simulink model "DOG_X_integer_true_two_paths_5b"  (R2024a)
settings: Solver=ode45  StartTime=0.0  StopTime=1.5*lsim*Ts  MaxStep=1/f0/2  RelTol=1e-6
values from neighbouring files (symbols this model uses):
  ft = (bint-1)*fbin    [exe_DOG_X_bit_true_2023a.m]    (also in exe_DOG_X_integer_true_two_paths_5b.m)
  g1 = g1_ideal*1    (= 4)    [exe_DOG_X_bit_true_2023a.m]    (also in exe_DOG_X_integer_true_two_paths_5b.m)
  Kvco = f0    (= 99840000)    [exe_DOG_X_bit_true_2023a.m]    (also in exe_DOG_X_integer_true_two_paths_5b.m)
  lvl = Vfs*10^(Input_signal_dB/20)    (= 0.125892541179)    [exe_DOG_X_bit_true_2023a.m]    (also in exe_DOG_X_integer_true_two_paths_5b.m)
  Nbsv1 = Nbvco+4    (= 9)    [exe_DOG_X_bit_true_2023a.m]    (also in exe_DOG_X_integer_true_two_paths_5b.m)
  Nbsv2 = Nbsv1+Nbext    [exe_DOG_X_bit_true_2023a.m]    (also in exe_DOG_X_integer_true_two_paths_5b.m)
  pnoi = 10^(-(60)/10)*(Vfs^2/2)    (= 5e-07)    [exe_DOG_X_bit_true_2023a.m]    (also in exe_DOG_X_integer_true_two_paths_5b.m)
  T2 = 1/f2    (= 4.06901041667e-08)    [exe_DOG_X_bit_true_2023a.m]    (also in exe_DOG_X_integer_true_two_paths_5b.m)
  Ts = 1/fs    (= 3.25520833333e-07)    [exe_DOG_X_bit_true_2023a.m]    (also in exe_DOG_X_integer_true_two_paths_5b.m)
  Tslow = 1/fslow    (= 6.51041666667e-07)    [exe_DOG_X_bit_true_2023a.m]    (also in exe_DOG_X_integer_true_two_paths_5b.m)
  Vfs = 1    [exe_DOG_X_bit_true_2023a.m]    (also in exe_DOG_X_integer_true_two_paths_5b.m)
undefined symbols (not defined in the file or in its folder): fa, fb, fti
libraries: simulink_extras x99, simulink x8
(part 1 of 4)
settings Model: SimulationMode=accelerator  Creator=lhernandez  LastModifiedBy=tremo
settings DataIOCC: SaveOutput=off  SignalLogging=off  DSMLogging=off  SaveTime=off  ReturnWorkspaceOutputs=off
settings RTWCC: GPUComputeCapability=3.5

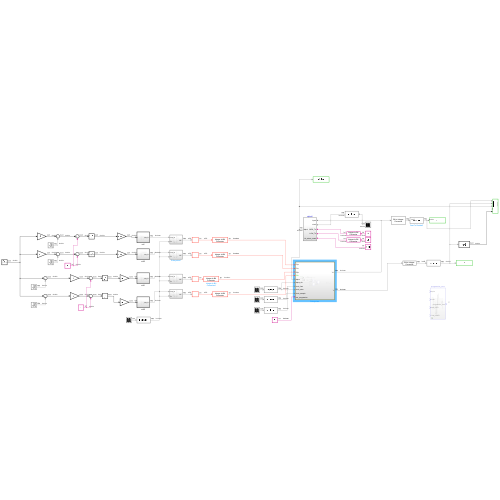
[thumbnail: Simulink's stored preview of the top-level diagram]
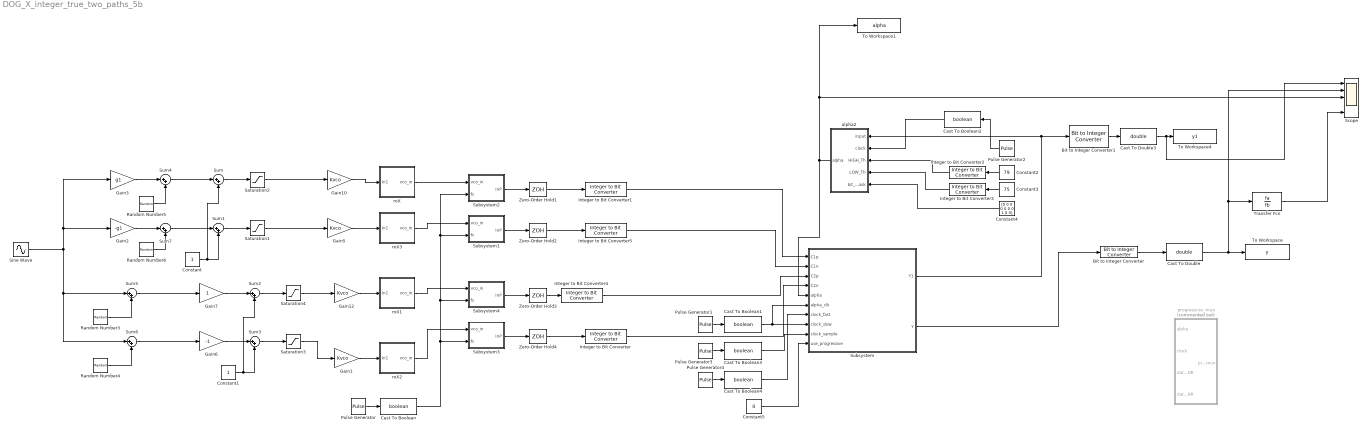
== system DOG_X_integer_true_two_paths_5b ==
  Bit to Integer Converter : simulink/Logic and Bit Operations/Bit to Integer Converter  nbits=11  bitOrder=MSB first  signedOutputValues=Signed  outDtype=Inherit via internal rule  outDtypeSigned=Inherit via internal rule
  Bit to Integer Converter1 : simulink/Logic and Bit Operations/Bit to Integer Converter  nbits=9  bitOrder=MSB first  signedOutputValues=Signed  outDtype=Inherit via internal rule  outDtypeSigned=Inherit via internal rule
  Cast To Boolean{,1..4} (5 alike) : DataTypeConversion  OutDataTypeStr=boolean  SaturateOnIntegerOverflow=off  RndMeth=Floor
  Cast To Double : DataTypeConversion  OutDataTypeStr=double  SaturateOnIntegerOverflow=off  RndMeth=Floor
  Cast To Double3 : DataTypeConversion  OutDataTypeStr=double  SaturateOnIntegerOverflow=off  RndMeth=Floor
  Constant : Constant
  Constant1 : Constant
  Constant2 : Constant  Value=79  OutDataTypeStr=fixdt(0,9,0)
  Constant3 : Constant  Value=75  OutDataTypeStr=fixdt(0,9,0)
  Constant4 : Constant  Value=[0 0 0 0 0 0 0 1 0 0]  OutDataTypeStr=boolean
  Constant5 : Constant  Value=0  OutDataTypeStr=boolean
  Gain{1,5,10,12} (4 alike) : Gain  Gain=Kvco
  Gain2 : Gain  Gain=-g1
  Gain3 : Gain  Gain=g1
  Gain6 : Gain  Gain=-1
  Gain7 : Gain
  Integer to Bit Converter{,1,4..5} (4 alike) : simulink/Logic and Bit Operations/Integer to Bit Converter  nbits=9  signedInputValues=Signed  bitOrder=MSB first  outDtype=boolean
  Integer to Bit Converter2 : simulink/Logic and Bit Operations/Integer to Bit Converter  nbits=9  signedInputValues=Unsigned  bitOrder=MSB first  outDtype=boolean
  Integer to Bit Converter3 : simulink/Logic and Bit Operations/Integer to Bit Converter  nbits=9  signedInputValues=Unsigned  bitOrder=MSB first  outDtype=boolean
  Pulse Generator : DiscretePulseGenerator  PulseType=Time based  Period=T2  PulseWidth=50
  Pulse Generator1 : DiscretePulseGenerator  PulseType=Time based  Period=Tslow  PulseWidth=50
  Pulse Generator2 : DiscretePulseGenerator  PulseType=Time based  Period=Tslow  PulseWidth=50
  Pulse Generator3 : DiscretePulseGenerator  PulseType=Time based  Period=Ts  PulseWidth=50
  Pulse Generator4 : DiscretePulseGenerator  PulseType=Time based  Period=T2  PulseWidth=50
  Random Number3 : RandomNumber  Variance=pnoi  Seed=35645  SampleTime=0
  Random Number4 : RandomNumber  Variance=pnoi  Seed=6854  SampleTime=0
  Random Number5 : RandomNumber  Variance=pnoi  Seed=5747  SampleTime=0
  Random Number6 : RandomNumber  Variance=pnoi  Seed=254745  SampleTime=0
  Saturation{1..4} (4 alike) : Saturate  UpperLimit=2  LowerLimit=0
  Scope : Scope  NumInputPorts=5
  Sine Wave : Sin  Amplitude=lvl/Vfs  Frequency=2*pi*ft  SampleTime=0
  Subsystem : Subsystem
  Subsystem1 : Subsystem
  Subsystem2 : Subsystem
  Subsystem3 : Subsystem
  Subsystem4 : Subsystem
  Sum{,1..7} (8 alike) : Sum  Inputs=|++
  To Workspace : ToWorkspace  VariableName=y  SampleTime=Ts
  To Workspace1 : ToWorkspace  VariableName=alpha  SampleTime=Ts
  To Workspace4 : ToWorkspace  VariableName=y1  SampleTime=Ts
  Transfer Fcn : TransferFcn  Numerator=fa  Denominator=fb
  Zero-Order Hold{1..4} (4 alike) : ZeroOrderHold  SampleTime=T2
  alpha2 : Subsystem
  progressive_mux : Subsystem  Commented=on
  roX : Subsystem
  roX1 : Subsystem
  roX2 : Subsystem
  roX3 : Subsystem
  wires:
  roX/1(vco_in) -> Subsystem2/1(vco_in)
  roX3/1(vco_in) -> Subsystem1/1(vco_in)
  Subsystem4/1(InP) -> Zero-Order Hold3/1
  Subsystem3/1(InP) -> Zero-Order Hold4/1
  Subsystem1/1(InP) -> Zero-Order Hold2/1
  Cast To Double/1 -> Transfer Fcn/1, Scope/2, To Workspace/1
  Cast To Double3/1 -> Scope/1, To Workspace4/1
  alpha2/1(alpha) -> Subsystem/5(alpha), To Workspace1/1, Scope/3
  Transfer Fcn/1 -> Scope/5
  Gain7/1 -> Sum2/1
  Saturation4/1 -> Gain12/1
  Sum5/1 -> Gain7/1
  Sum7/1 -> Sum1/1
  Gain10/1 -> roX/1(In1)
  Sum4/1 -> Sum/1
  Random Number6/1 -> Sum7/2
  Random Number4/1 -> Sum6/2
  Random Number3/1 -> Sum5/2
  Sine Wave/1 -> Sum6/1, Sum5/1, Gain3/1, Gain2/1
  Constant1/1 -> Sum2/2, Sum3/2
  Sum6/1 -> Gain6/1
  Sum/1 -> Saturation2/1
  Sum3/1 -> Saturation3/1
  Constant/1 -> Sum/2, Sum1/2
  Gain5/1 -> roX3/1(In1)
  Random Number5/1 -> Sum4/2
  Gain3/1 -> Sum4/1
  Gain2/1 -> Sum7/1
  Saturation3/1 -> Gain1/1
  Saturation2/1 -> Gain10/1
  Sum1/1 -> Saturation1/1
  Gain12/1 -> roX1/1(In1)
  Gain6/1 -> Sum3/1
  Sum2/1 -> Saturation4/1
  Saturation1/1 -> Gain5/1
  Gain1/1 -> roX2/1(In1)
  Subsystem2/1(InP) -> Zero-Order Hold1/1
  roX1/1(vco_in) -> Subsystem4/1(vco_in)
  roX2/1(vco_in) -> Subsystem3/1(vco_in)
  Zero-Order Hold3/1 -> Integer to Bit Converter4/1
  Zero-Order Hold4/1 -> Integer to Bit Converter/1
  Pulse Generator/1 -> Cast To Boolean/1
  Cast To Boolean/1 -> Subsystem3/2(fs), Subsystem4/2(fs), Subsystem1/2(fs), Subsystem2/2(fs)
  Subsystem/1(Y1) -> Bit to Integer Converter1/1, alpha2/1(input)
  Pulse Generator2/1 -> Cast To Boolean2/1
  Cast To Boolean2/1 -> alpha2/2(clock)
  Constant2/1 -> Integer to Bit Converter2/1
  Integer to Bit Converter2/1 -> alpha2/3(HIGH_Th)
  Constant3/1 -> Integer to Bit Converter3/1
  Integer to Bit Converter3/1 -> alpha2/4(LOW_Th)
  Constant4/1 -> alpha2/5(bit_select_mask)
  Bit to Integer Converter/1 -> Cast To Double/1
  Pulse Generator1/1 -> Cast To Boolean1/1
  Cast To Boolean1/1 -> Subsystem/8(clock_slow), Subsystem/6(alpha_clk)
  Integer to Bit Converter/1 -> Subsystem/4(C2n)
  Integer to Bit Converter4/1 -> Subsystem/3(C2p)
  Zero-Order Hold2/1 -> Integer to Bit Converter5/1
  Zero-Order Hold1/1 -> Integer to Bit Converter1/1
  Pulse Generator3/1 -> Cast To Boolean3/1
  Cast To Boolean3/1 -> Subsystem/9(clock_sample)
  Pulse Generator4/1 -> Cast To Boolean4/1
  Cast To Boolean4/1 -> Subsystem/7(clock_fast)
  Bit to Integer Converter1/1 -> Cast To Double3/1
  Integer to Bit Converter1/1 -> Subsystem/1(C1p)
  Integer to Bit Converter5/1 -> Subsystem/2(C1n)
  Subsystem/2(Y) -> Bit to Integer Converter/1
  Constant5/1 -> Subsystem/10(use_progressive)

== system DOG_X_integer_true_two_paths_5b/Subsystem ==
  C1p : Inport
  C1n : Inport  Port=2
  C2p : Inport  Port=3
  C2n : Inport  Port=4
  alpha : Inport  Port=5
  alpha_clk : Inport  Port=6
  clock_fast : Inport  Port=7
  clock_slow : Inport  Port=8
  clock_sample : Inport  Port=9
  use_progressive : Inport  Port=10
  " 2 bit arithmetic left shift" : Subsystem
  " 2 bit extension" : Subsystem
  2ND_Noise_Shaper_pipelined3 : Subsystem
  Noise_shaper1 : Subsystem
  Noise_shaper2 : Subsystem
  Terminator : Terminator
  mux : Subsystem
  mux1 : Subsystem
  progressive_mux : Subsystem
  substractor2 : Subsystem
  Y1 : Outport
  Y : Outport  Port=2
  wires:
  Noise_shaper2/2(Y1) -> Y1/1
  substractor2/1(Cmux1) -> 2ND_Noise_Shaper_pipelined3/1(Cmux1)
  C2p/1 -> Noise_shaper2/1(InP)
  C2n/1 -> Noise_shaper2/2(InN)
  alpha_clk/1 -> progressive_mux/4(clock)
  alpha/1 -> mux/3(alpha), progressive_mux/3(alpha)
  progressive_mux/1(progressive_mux) -> mux1/1(progressive)
  clock_fast/1 -> Noise_shaper1/3(clock_fast), Noise_shaper2/3(clock_fast)
  clock_slow/1 -> Noise_shaper1/4(clock_slow), Noise_shaper2/4(clock_slow)
  Noise_shaper2/1(Y) -> " 2 bit arithmetic left shift"/1(in)
  " 2 bit arithmetic left shift"/1(x4) -> mux/1(data_HDR), progressive_mux/1(data_HDR)
  clock_sample/1 -> Noise_shaper1/5(clock_sample), Noise_shaper2/5(clock_sample)
  " 2 bit extension"/1(extended) -> mux/2(data_HSNR), progressive_mux/2(data_HSNR)
  C1n/1 -> Noise_shaper1/2(InN)
  C1p/1 -> Noise_shaper1/1(InP)
  Noise_shaper1/1(Y) -> " 2 bit extension"/1(in)
  Noise_shaper1/2(Y1) -> Terminator/1
  mux/1(out) -> mux1/2(non_progressive)
  mux1/1(out) -> Y/1
  use_progressive/1 -> mux1/3(select)

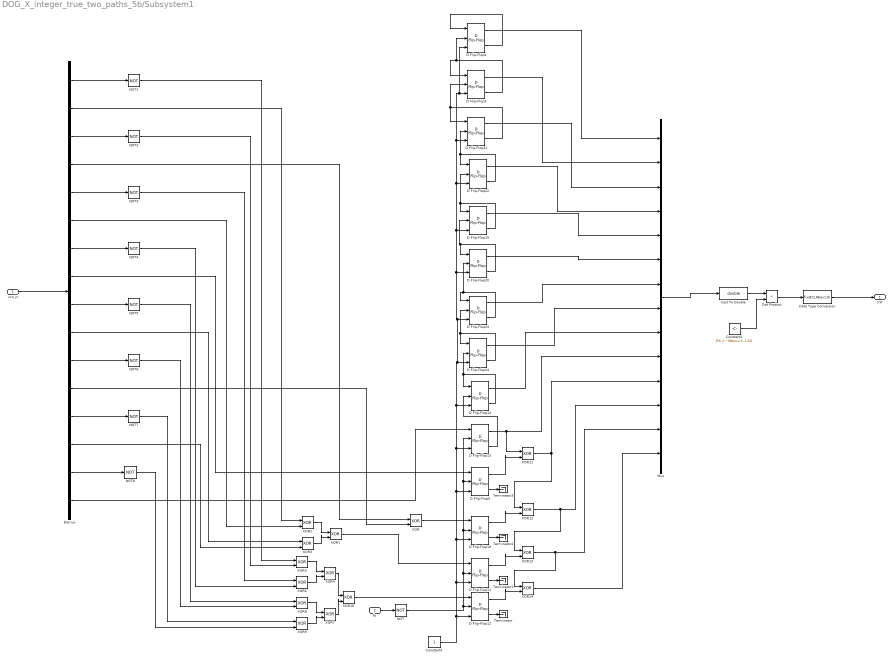
== system DOG_X_integer_true_two_paths_5b/Subsystem1 ==
  vco_in : Inport
  fs : Inport  Port=2
  Cast To Double : DataTypeConversion  OutDataTypeStr=double  SaturateOnIntegerOverflow=off  RndMeth=Floor
  Constant1 : Constant  Value=[fti 2.^(Nbsv1-1:-1:0)]
  Constant4 : Constant
  D Flip-Flop{3..4,9..15,20..24} (14 alike) : simulink_extras/Flip Flops/D Flip-Flop
  Data Type Conversion : DataTypeConversion  OutDataTypeStr=fixdt(1,Nbsv1,0)  SaturateOnIntegerOverflow=off  RndMeth=Floor
  Demux : Demux  Outputs=16
  Dot Product : DotProduct  OutDataTypeStr=Inherit: Inherit via internal rule
  Mux : Mux  Inputs=14
  NOT{,1..8} (9 alike) : Logic  Operator=NOT  IconShape=distinctive  AllPortsSameDT=off  OutDataTypeStr=boolean
  Terminator{,1..3} (4 alike) : Terminator
  XOR{,1..14} (15 alike) : Logic  Operator=XOR  IconShape=distinctive  AllPortsSameDT=off  OutDataTypeStr=boolean
  InP : Outport
  wires:
  D Flip-Flop12/2 -> Terminator/1
  D Flip-Flop10/2 -> Terminator2/1
  D Flip-Flop11/2 -> Terminator1/1
  D Flip-Flop22/2 -> D Flip-Flop21/2, D Flip-Flop22/1
  D Flip-Flop21/2 -> D Flip-Flop21/1, D Flip-Flop3/2
  D Flip-Flop23/2 -> D Flip-Flop20/2, D Flip-Flop23/1
  D Flip-Flop24/2 -> D Flip-Flop24/1, D Flip-Flop23/2
  D Flip-Flop20/2 -> D Flip-Flop15/2, D Flip-Flop20/1
  D Flip-Flop15/2 -> D Flip-Flop22/2, D Flip-Flop15/1
  Dot Product/1 -> Data Type Conversion/1
  Cast To Double/1 -> Dot Product/1
  Mux/1 -> Cast To Double/1
  fs/1 -> NOT/1
  D Flip-Flop14/2 -> D Flip-Flop14/1, D Flip-Flop24/2
  Constant1/1 -> Dot Product/2
  Data Type Conversion/1 -> InP/1
  Constant4/1 -> D Flip-Flop12/3, D Flip-Flop11/3, D Flip-Flop10/3, D Flip-Flop4/3, D Flip-Flop3/3, D Flip-Flop21/3, D Flip-Flop22/3, D Flip-Flop15/3, D Flip-Flop20/3, D Flip-Flop23/3, D Flip-Flop24/3, D Flip-Flop14/3, D Flip-Flop13/3, D Flip-Flop9/3
  D Flip-Flop13/2 -> D Flip-Flop14/2
  NOT/1 -> D Flip-Flop12/2, D Flip-Flop13/2, D Flip-Flop9/2, D Flip-Flop10/2, D Flip-Flop11/2
  D Flip-Flop3/2 -> D Flip-Flop4/2, D Flip-Flop3/1
  D Flip-Flop4/2 -> D Flip-Flop4/1
  D Flip-Flop4/1 -> Mux/1
  D Flip-Flop3/1 -> Mux/2
  D Flip-Flop21/1 -> Mux/3
  D Flip-Flop22/1 -> Mux/4
  D Flip-Flop15/1 -> Mux/5
  D Flip-Flop20/1 -> Mux/6
  D Flip-Flop23/1 -> Mux/7
  D Flip-Flop24/1 -> Mux/8
  D Flip-Flop14/1 -> Mux/9
  D Flip-Flop9/2 -> Terminator3/1
  vco_in/1 -> Demux/1
  Demux/1 -> NOT1/1
  Demux/5 -> NOT3/1
  Demux/7 -> NOT4/1
  Demux/9 -> NOT5/1
  Demux/13 -> NOT7/1
  Demux/15 -> NOT8/1
  Demux/11 -> NOT6/1
  Demux/4 -> XOR/1
  Demux/12 -> XOR/2
  XOR2/1 -> XOR1/1
  XOR3/1 -> XOR1/2
  Demux/2 -> XOR2/1
  Demux/6 -> XOR2/2
  Demux/10 -> XOR3/1
  Demux/14 -> XOR3/2
  XOR5/1 -> XOR4/1
  XOR6/1 -> XOR4/2
  XOR8/1 -> XOR7/1
  XOR9/1 -> XOR7/2
  XOR4/1 -> XOR10/1
  XOR7/1 -> XOR10/2
  Demux/3 -> NOT2/1
  D Flip-Flop13/1 -> XOR11/1, Mux/10
  D Flip-Flop9/1 -> XOR11/2
  XOR11/1 -> Mux/11, XOR12/1
  D Flip-Flop10/1 -> XOR12/2
  XOR12/1 -> XOR13/1, Mux/12
  D Flip-Flop11/1 -> XOR13/2
  XOR13/1 -> XOR14/1, Mux/13
  D Flip-Flop12/1 -> XOR14/2
  XOR14/1 -> Mux/14
  NOT1/1 -> XOR5/1
  NOT2/1 -> XOR5/2
  NOT3/1 -> XOR6/1
  NOT4/1 -> XOR6/2
  NOT5/1 -> XOR8/1
  NOT6/1 -> XOR8/2
  NOT7/1 -> XOR9/1
  NOT8/1 -> XOR9/2
  Demux/16 -> D Flip-Flop13/1
  Demux/8 -> D Flip-Flop9/1
  XOR/1 -> D Flip-Flop10/1
  XOR1/1 -> D Flip-Flop11/1
  XOR10/1 -> D Flip-Flop12/1

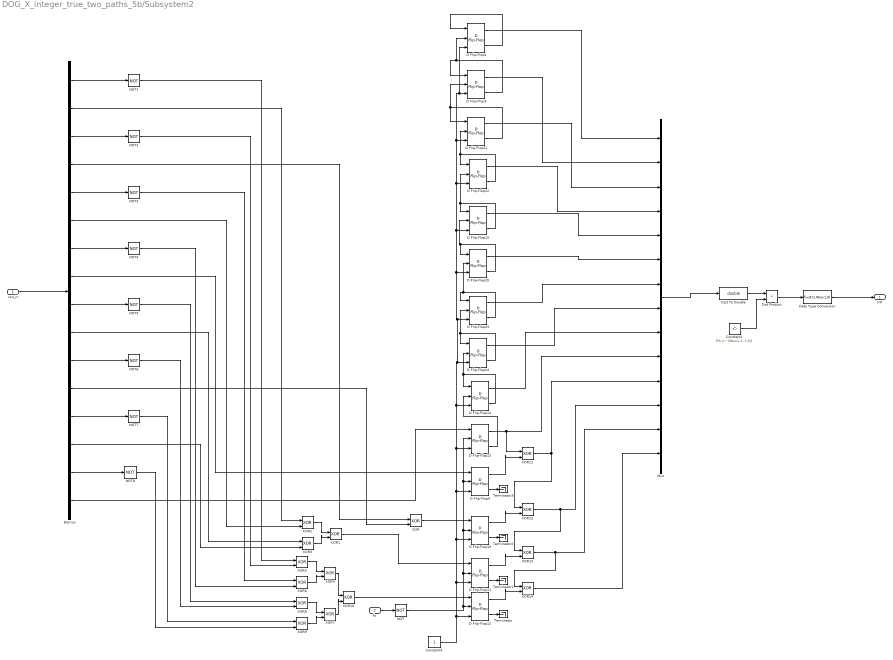
== system DOG_X_integer_true_two_paths_5b/Subsystem2 ==
  vco_in : Inport
  fs : Inport  Port=2
  Cast To Double : DataTypeConversion  OutDataTypeStr=double  SaturateOnIntegerOverflow=off  RndMeth=Floor
  Constant1 : Constant  Value=[fti 2.^(Nbsv1-1:-1:0)]
  Constant4 : Constant
  D Flip-Flop{3..4,9..15,20..24} (14 alike) : simulink_extras/Flip Flops/D Flip-Flop
  Data Type Conversion : DataTypeConversion  OutDataTypeStr=fixdt(1,Nbsv1,0)  SaturateOnIntegerOverflow=off  RndMeth=Floor
  Demux : Demux  Outputs=16
  Dot Product : DotProduct  OutDataTypeStr=Inherit: Inherit via internal rule
  Mux : Mux  Inputs=14
  NOT{,1..8} (9 alike) : Logic  Operator=NOT  IconShape=distinctive  AllPortsSameDT=off  OutDataTypeStr=boolean
  Terminator{,1..3} (4 alike) : Terminator
  XOR{,1..14} (15 alike) : Logic  Operator=XOR  IconShape=distinctive  AllPortsSameDT=off  OutDataTypeStr=boolean
  InP : Outport
  wires:
  D Flip-Flop12/2 -> Terminator/1
  D Flip-Flop10/2 -> Terminator2/1
  D Flip-Flop11/2 -> Terminator1/1
  D Flip-Flop22/2 -> D Flip-Flop21/2, D Flip-Flop22/1
  D Flip-Flop21/2 -> D Flip-Flop21/1, D Flip-Flop3/2
  D Flip-Flop23/2 -> D Flip-Flop20/2, D Flip-Flop23/1
  D Flip-Flop24/2 -> D Flip-Flop24/1, D Flip-Flop23/2
  D Flip-Flop20/2 -> D Flip-Flop15/2, D Flip-Flop20/1
  D Flip-Flop15/2 -> D Flip-Flop22/2, D Flip-Flop15/1
  Dot Product/1 -> Data Type Conversion/1
  Cast To Double/1 -> Dot Product/1
  Mux/1 -> Cast To Double/1
  fs/1 -> NOT/1
  D Flip-Flop14/2 -> D Flip-Flop14/1, D Flip-Flop24/2
  Constant1/1 -> Dot Product/2
  Data Type Conversion/1 -> InP/1
  Constant4/1 -> D Flip-Flop12/3, D Flip-Flop11/3, D Flip-Flop10/3, D Flip-Flop4/3, D Flip-Flop3/3, D Flip-Flop21/3, D Flip-Flop22/3, D Flip-Flop15/3, D Flip-Flop20/3, D Flip-Flop23/3, D Flip-Flop24/3, D Flip-Flop14/3, D Flip-Flop13/3, D Flip-Flop9/3
  D Flip-Flop13/2 -> D Flip-Flop14/2
  NOT/1 -> D Flip-Flop12/2, D Flip-Flop13/2, D Flip-Flop9/2, D Flip-Flop10/2, D Flip-Flop11/2
  D Flip-Flop3/2 -> D Flip-Flop4/2, D Flip-Flop3/1
  D Flip-Flop4/2 -> D Flip-Flop4/1
  D Flip-Flop4/1 -> Mux/1
  D Flip-Flop3/1 -> Mux/2
  D Flip-Flop21/1 -> Mux/3
  D Flip-Flop22/1 -> Mux/4
  D Flip-Flop15/1 -> Mux/5
  D Flip-Flop20/1 -> Mux/6
  D Flip-Flop23/1 -> Mux/7
  D Flip-Flop24/1 -> Mux/8
  D Flip-Flop14/1 -> Mux/9
  D Flip-Flop9/2 -> Terminator3/1
  vco_in/1 -> Demux/1
  Demux/1 -> NOT1/1
  Demux/5 -> NOT3/1
  Demux/7 -> NOT4/1
  Demux/9 -> NOT5/1
  Demux/13 -> NOT7/1
  Demux/15 -> NOT8/1
  Demux/11 -> NOT6/1
  Demux/4 -> XOR/1
  Demux/12 -> XOR/2
  XOR2/1 -> XOR1/1
  XOR3/1 -> XOR1/2
  Demux/2 -> XOR2/1
  Demux/6 -> XOR2/2
  Demux/10 -> XOR3/1
  Demux/14 -> XOR3/2
  XOR5/1 -> XOR4/1
  XOR6/1 -> XOR4/2
  XOR8/1 -> XOR7/1
  XOR9/1 -> XOR7/2
  XOR4/1 -> XOR10/1
  XOR7/1 -> XOR10/2
  Demux/3 -> NOT2/1
  D Flip-Flop13/1 -> XOR11/1, Mux/10
  D Flip-Flop9/1 -> XOR11/2
  XOR11/1 -> Mux/11, XOR12/1
  D Flip-Flop10/1 -> XOR12/2
  XOR12/1 -> XOR13/1, Mux/12
  D Flip-Flop11/1 -> XOR13/2
  XOR13/1 -> XOR14/1, Mux/13
  D Flip-Flop12/1 -> XOR14/2
  XOR14/1 -> Mux/14
  NOT1/1 -> XOR5/1
  NOT2/1 -> XOR5/2
  NOT3/1 -> XOR6/1
  NOT4/1 -> XOR6/2
  NOT5/1 -> XOR8/1
  NOT6/1 -> XOR8/2
  NOT7/1 -> XOR9/1
  NOT8/1 -> XOR9/2
  Demux/16 -> D Flip-Flop13/1
  Demux/8 -> D Flip-Flop9/1
  XOR/1 -> D Flip-Flop10/1
  XOR1/1 -> D Flip-Flop11/1
  XOR10/1 -> D Flip-Flop12/1

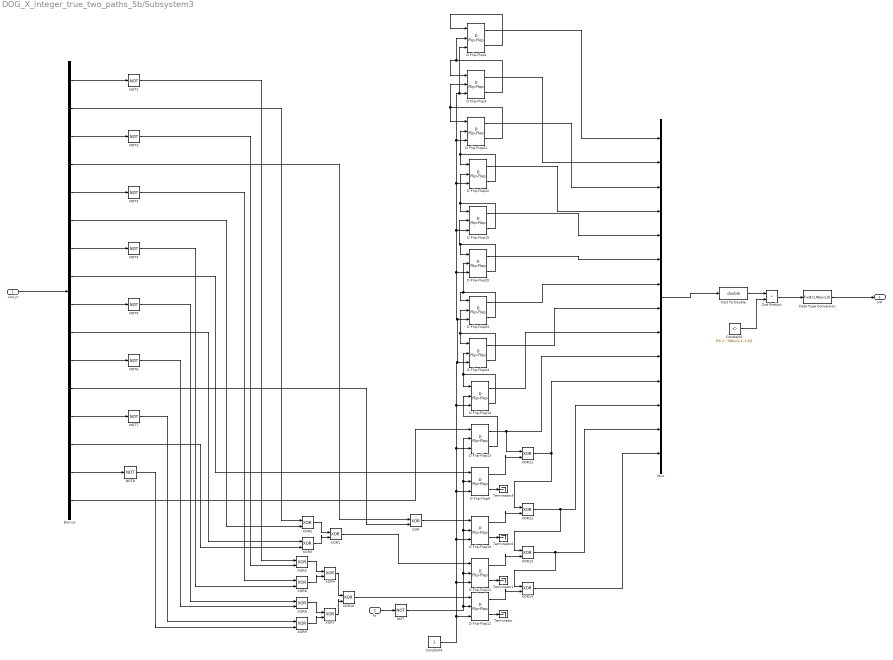
== system DOG_X_integer_true_two_paths_5b/Subsystem3 ==
  vco_in : Inport
  fs : Inport  Port=2
  Cast To Double : DataTypeConversion  OutDataTypeStr=double  SaturateOnIntegerOverflow=off  RndMeth=Floor
  Constant1 : Constant  Value=[fti 2.^(Nbsv1-1:-1:0)]
  Constant4 : Constant
  D Flip-Flop{3..4,9..15,20..24} (14 alike) : simulink_extras/Flip Flops/D Flip-Flop
  Data Type Conversion : DataTypeConversion  OutDataTypeStr=fixdt(1,Nbsv1,0)  SaturateOnIntegerOverflow=off  RndMeth=Floor
  Demux : Demux  Outputs=16
  Dot Product : DotProduct  OutDataTypeStr=Inherit: Inherit via internal rule
  Mux : Mux  Inputs=14
  NOT{,1..8} (9 alike) : Logic  Operator=NOT  IconShape=distinctive  AllPortsSameDT=off  OutDataTypeStr=boolean
  Terminator{,1..3} (4 alike) : Terminator
  XOR{,1..14} (15 alike) : Logic  Operator=XOR  IconShape=distinctive  AllPortsSameDT=off  OutDataTypeStr=boolean
  InP : Outport
  wires:
  D Flip-Flop12/2 -> Terminator/1
  D Flip-Flop10/2 -> Terminator2/1
  D Flip-Flop11/2 -> Terminator1/1
  D Flip-Flop22/2 -> D Flip-Flop21/2, D Flip-Flop22/1
  D Flip-Flop21/2 -> D Flip-Flop21/1, D Flip-Flop3/2
  D Flip-Flop23/2 -> D Flip-Flop20/2, D Flip-Flop23/1
  D Flip-Flop24/2 -> D Flip-Flop24/1, D Flip-Flop23/2
  D Flip-Flop20/2 -> D Flip-Flop15/2, D Flip-Flop20/1
  D Flip-Flop15/2 -> D Flip-Flop22/2, D Flip-Flop15/1
  Dot Product/1 -> Data Type Conversion/1
  Cast To Double/1 -> Dot Product/1
  Mux/1 -> Cast To Double/1
  fs/1 -> NOT/1
  D Flip-Flop14/2 -> D Flip-Flop14/1, D Flip-Flop24/2
  Constant1/1 -> Dot Product/2
  Data Type Conversion/1 -> InP/1
  Constant4/1 -> D Flip-Flop12/3, D Flip-Flop11/3, D Flip-Flop10/3, D Flip-Flop4/3, D Flip-Flop3/3, D Flip-Flop21/3, D Flip-Flop22/3, D Flip-Flop15/3, D Flip-Flop20/3, D Flip-Flop23/3, D Flip-Flop24/3, D Flip-Flop14/3, D Flip-Flop13/3, D Flip-Flop9/3
  D Flip-Flop13/2 -> D Flip-Flop14/2
  NOT/1 -> D Flip-Flop12/2, D Flip-Flop13/2, D Flip-Flop9/2, D Flip-Flop10/2, D Flip-Flop11/2
  D Flip-Flop3/2 -> D Flip-Flop4/2, D Flip-Flop3/1
  D Flip-Flop4/2 -> D Flip-Flop4/1
  D Flip-Flop4/1 -> Mux/1
  D Flip-Flop3/1 -> Mux/2
  D Flip-Flop21/1 -> Mux/3
  D Flip-Flop22/1 -> Mux/4
  D Flip-Flop15/1 -> Mux/5
  D Flip-Flop20/1 -> Mux/6
  D Flip-Flop23/1 -> Mux/7
  D Flip-Flop24/1 -> Mux/8
  D Flip-Flop14/1 -> Mux/9
  D Flip-Flop9/2 -> Terminator3/1
  vco_in/1 -> Demux/1
  Demux/1 -> NOT1/1
  Demux/5 -> NOT3/1
  Demux/7 -> NOT4/1
  Demux/9 -> NOT5/1
  Demux/13 -> NOT7/1
  Demux/15 -> NOT8/1
  Demux/11 -> NOT6/1
  Demux/4 -> XOR/1
  Demux/12 -> XOR/2
  XOR2/1 -> XOR1/1
  XOR3/1 -> XOR1/2
  Demux/2 -> XOR2/1
  Demux/6 -> XOR2/2
  Demux/10 -> XOR3/1
  Demux/14 -> XOR3/2
  XOR5/1 -> XOR4/1
  XOR6/1 -> XOR4/2
  XOR8/1 -> XOR7/1
  XOR9/1 -> XOR7/2
  XOR4/1 -> XOR10/1
  XOR7/1 -> XOR10/2
  Demux/3 -> NOT2/1
  D Flip-Flop13/1 -> XOR11/1, Mux/10
  D Flip-Flop9/1 -> XOR11/2
  XOR11/1 -> Mux/11, XOR12/1
  D Flip-Flop10/1 -> XOR12/2
  XOR12/1 -> XOR13/1, Mux/12
  D Flip-Flop11/1 -> XOR13/2
  XOR13/1 -> XOR14/1, Mux/13
  D Flip-Flop12/1 -> XOR14/2
  XOR14/1 -> Mux/14
  NOT1/1 -> XOR5/1
  NOT2/1 -> XOR5/2
  NOT3/1 -> XOR6/1
  NOT4/1 -> XOR6/2
  NOT5/1 -> XOR8/1
  NOT6/1 -> XOR8/2
  NOT7/1 -> XOR9/1
  NOT8/1 -> XOR9/2
  Demux/16 -> D Flip-Flop13/1
  Demux/8 -> D Flip-Flop9/1
  XOR/1 -> D Flip-Flop10/1
  XOR1/1 -> D Flip-Flop11/1
  XOR10/1 -> D Flip-Flop12/1

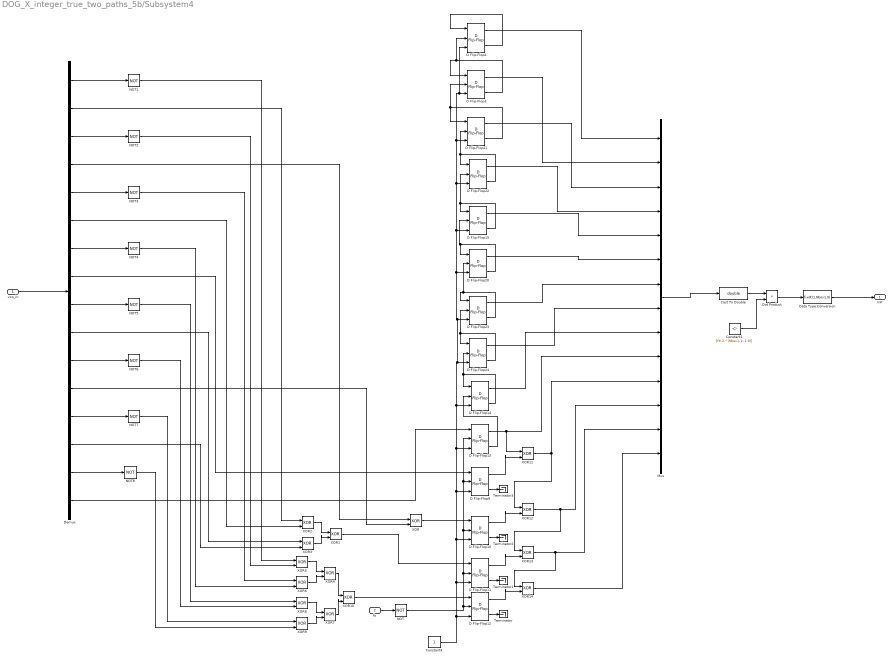
== system DOG_X_integer_true_two_paths_5b/Subsystem4 ==
  vco_in : Inport
  fs : Inport  Port=2
  Cast To Double : DataTypeConversion  OutDataTypeStr=double  SaturateOnIntegerOverflow=off  RndMeth=Floor
  Constant1 : Constant  Value=[fti 2.^(Nbsv1-1:-1:0)]
  Constant4 : Constant
  D Flip-Flop{3..4,9..15,20..24} (14 alike) : simulink_extras/Flip Flops/D Flip-Flop
  Data Type Conversion : DataTypeConversion  OutDataTypeStr=fixdt(1,Nbsv1,0)  SaturateOnIntegerOverflow=off  RndMeth=Floor
  Demux : Demux  Outputs=16
  Dot Product : DotProduct  OutDataTypeStr=Inherit: Inherit via internal rule
  Mux : Mux  Inputs=14
  NOT{,1..8} (9 alike) : Logic  Operator=NOT  IconShape=distinctive  AllPortsSameDT=off  OutDataTypeStr=boolean
  Terminator{,1..3} (4 alike) : Terminator
  XOR{,1..14} (15 alike) : Logic  Operator=XOR  IconShape=distinctive  AllPortsSameDT=off  OutDataTypeStr=boolean
  InP : Outport
  wires:
  D Flip-Flop12/2 -> Terminator/1
  D Flip-Flop10/2 -> Terminator2/1
  D Flip-Flop11/2 -> Terminator1/1
  D Flip-Flop22/2 -> D Flip-Flop21/2, D Flip-Flop22/1
  D Flip-Flop21/2 -> D Flip-Flop21/1, D Flip-Flop3/2
  D Flip-Flop23/2 -> D Flip-Flop20/2, D Flip-Flop23/1
  D Flip-Flop24/2 -> D Flip-Flop24/1, D Flip-Flop23/2
  D Flip-Flop20/2 -> D Flip-Flop15/2, D Flip-Flop20/1
  D Flip-Flop15/2 -> D Flip-Flop22/2, D Flip-Flop15/1
  Dot Product/1 -> Data Type Conversion/1
  Cast To Double/1 -> Dot Product/1
  Mux/1 -> Cast To Double/1
  fs/1 -> NOT/1
  D Flip-Flop14/2 -> D Flip-Flop14/1, D Flip-Flop24/2
  Constant1/1 -> Dot Product/2
  Data Type Conversion/1 -> InP/1
  Constant4/1 -> D Flip-Flop12/3, D Flip-Flop11/3, D Flip-Flop10/3, D Flip-Flop4/3, D Flip-Flop3/3, D Flip-Flop21/3, D Flip-Flop22/3, D Flip-Flop15/3, D Flip-Flop20/3, D Flip-Flop23/3, D Flip-Flop24/3, D Flip-Flop14/3, D Flip-Flop13/3, D Flip-Flop9/3
  D Flip-Flop13/2 -> D Flip-Flop14/2
  NOT/1 -> D Flip-Flop12/2, D Flip-Flop13/2, D Flip-Flop9/2, D Flip-Flop10/2, D Flip-Flop11/2
  D Flip-Flop3/2 -> D Flip-Flop4/2, D Flip-Flop3/1
  D Flip-Flop4/2 -> D Flip-Flop4/1
  D Flip-Flop4/1 -> Mux/1
  D Flip-Flop3/1 -> Mux/2
  D Flip-Flop21/1 -> Mux/3
  D Flip-Flop22/1 -> Mux/4
  D Flip-Flop15/1 -> Mux/5
  D Flip-Flop20/1 -> Mux/6
  D Flip-Flop23/1 -> Mux/7
  D Flip-Flop24/1 -> Mux/8
  D Flip-Flop14/1 -> Mux/9
  D Flip-Flop9/2 -> Terminator3/1
  vco_in/1 -> Demux/1
  Demux/1 -> NOT1/1
  Demux/5 -> NOT3/1
  Demux/7 -> NOT4/1
  Demux/9 -> NOT5/1
  Demux/13 -> NOT7/1
  Demux/15 -> NOT8/1
  Demux/11 -> NOT6/1
  Demux/4 -> XOR/1
  Demux/12 -> XOR/2
  XOR2/1 -> XOR1/1
  XOR3/1 -> XOR1/2
  Demux/2 -> XOR2/1
  Demux/6 -> XOR2/2
  Demux/10 -> XOR3/1
  Demux/14 -> XOR3/2
  XOR5/1 -> XOR4/1
  XOR6/1 -> XOR4/2
  XOR8/1 -> XOR7/1
  XOR9/1 -> XOR7/2
  XOR4/1 -> XOR10/1
  XOR7/1 -> XOR10/2
  Demux/3 -> NOT2/1
  D Flip-Flop13/1 -> XOR11/1, Mux/10
  D Flip-Flop9/1 -> XOR11/2
  XOR11/1 -> Mux/11, XOR12/1
  D Flip-Flop10/1 -> XOR12/2
  XOR12/1 -> XOR13/1, Mux/12
  D Flip-Flop11/1 -> XOR13/2
  XOR13/1 -> XOR14/1, Mux/13
  D Flip-Flop12/1 -> XOR14/2
  XOR14/1 -> Mux/14
  NOT1/1 -> XOR5/1
  NOT2/1 -> XOR5/2
  NOT3/1 -> XOR6/1
  NOT4/1 -> XOR6/2
  NOT5/1 -> XOR8/1
  NOT6/1 -> XOR8/2
  NOT7/1 -> XOR9/1
  NOT8/1 -> XOR9/2
  Demux/16 -> D Flip-Flop13/1
  Demux/8 -> D Flip-Flop9/1
  XOR/1 -> D Flip-Flop10/1
  XOR1/1 -> D Flip-Flop11/1
  XOR10/1 -> D Flip-Flop12/1

== system DOG_X_integer_true_two_paths_5b/alpha2 ==
  note: si a > b, reset
  note: si a > b, HDR
  input : Inport
  clock : Inport  Port=2
  HIGH_Th : Inport  Port=3
  LOW_Th : Inport  Port=4
  bit_select_mask : Inport  Port=5
  10 bit  counter (pos) : Subsystem
  AND : Logic  IconShape=distinctive  AllPortsSameDT=off  OutDataTypeStr=boolean
  AND1 : Logic  IconShape=distinctive  AllPortsSameDT=off  OutDataTypeStr=boolean
  NOT : Logic  Operator=NOT  IconShape=distinctive  AllPortsSameDT=off  OutDataTypeStr=boolean
  NOT1 : Logic  Operator=NOT  IconShape=distinctive  AllPortsSameDT=off  OutDataTypeStr=boolean
  NOT2 : Logic  Operator=NOT  IconShape=distinctive  AllPortsSameDT=off  OutDataTypeStr=boolean
  S-R Flip-Flop : simulink_extras/Flip Flops/S-R Flip-Flop  initial_condition=0
  Terminator : Terminator
  abs : Subsystem
  comp_HI_Threshold : Subsystem
  comp_LOW_Threshold : Subsystem
  alpha : Outport
  wires:
  input/1 -> abs/1(input)
  S-R Flip-Flop/1 -> alpha/1
  clock/1 -> 10 bit  counter (pos)/2(clock)
  LOW_Th/1 -> comp_LOW_Threshold/2(b)
  NOT1/1 -> 10 bit  counter (pos)/3(!reset)
  abs/1(abs(input)) -> comp_HI_Threshold/1(a), comp_LOW_Threshold/1(a)
  HIGH_Th/1 -> comp_HI_Threshold/2(b)
  S-R Flip-Flop/2 -> Terminator/1
  comp_LOW_Threshold/1(a < b) -> AND/2
  AND1/1 -> S-R Flip-Flop/2
  comp_HI_Threshold/1(a > b) -> NOT1/1, NOT2/1, S-R Flip-Flop/1
  NOT/1 -> AND/1
  NOT2/1 -> AND1/1
  10 bit  counter (pos)/1(count_selected_bit) -> AND1/2, NOT/1
  AND/1 -> 10 bit  counter (pos)/1(count_enable)
  bit_select_mask/1 -> 10 bit  counter (pos)/4(bit_select_mask)

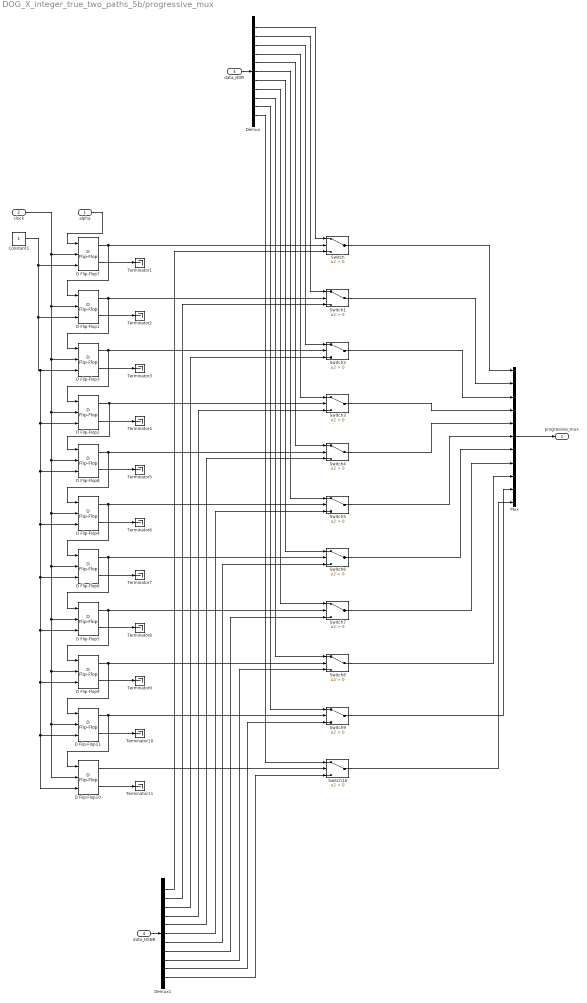
== system DOG_X_integer_true_two_paths_5b/progressive_mux ==
  alpha : Inport
  clock : Inport  Port=2
  data_HDR : Inport  Port=3
  data_HSNR : Inport  Port=4
  Constant1 : Constant  OutDataTypeStr=boolean
  D Flip-Flop{1..11} (11 alike) : simulink_extras/Flip Flops/D Flip-Flop
  Demux : Demux  Outputs=11
  Demux1 : Demux  Outputs=11
  Mux : Mux  Inputs=11
  Switch{,1..10} (11 alike) : Switch  Criteria=u2 > Threshold  SaturateOnIntegerOverflow=off  InputSameDT=off
  Terminator{1..11} (11 alike) : Terminator
  progressive_mux : Outport
  wires:
  D Flip-Flop7/1 -> Switch/2, D Flip-Flop1/1
  data_HDR/1 -> Demux/1
  data_HSNR/1 -> Demux1/1
  D Flip-Flop7/2 -> Terminator1/1
  D Flip-Flop1/2 -> Terminator2/1
  D Flip-Flop1/1 -> D Flip-Flop3/1, Switch1/2
  D Flip-Flop3/1 -> Switch2/2, D Flip-Flop2/1
  D Flip-Flop2/2 -> Terminator4/1
  D Flip-Flop3/2 -> Terminator3/1
  D Flip-Flop2/1 -> Switch3/2, D Flip-Flop8/1
  D Flip-Flop4/2 -> Terminator6/1
  D Flip-Flop8/1 -> Switch4/2, D Flip-Flop4/1
  D Flip-Flop6/2 -> Terminator7/1
  D Flip-Flop5/2 -> Terminator8/1
  D Flip-Flop6/1 -> Switch6/2, D Flip-Flop5/1
  D Flip-Flop8/2 -> Terminator5/1
  D Flip-Flop4/1 -> D Flip-Flop6/1, Switch5/2
  D Flip-Flop11/1 -> Switch9/2, D Flip-Flop10/1
  D Flip-Flop9/1 -> D Flip-Flop11/1, Switch8/2
  D Flip-Flop5/1 -> D Flip-Flop9/1, Switch7/2
  D Flip-Flop9/2 -> Terminator9/1
  D Flip-Flop11/2 -> Terminator10/1
  D Flip-Flop10/1 -> Switch10/2
  Constant1/1 -> D Flip-Flop8/3, D Flip-Flop10/3, D Flip-Flop11/3, D Flip-Flop9/3, D Flip-Flop5/3, D Flip-Flop6/3, D Flip-Flop4/3, D Flip-Flop2/3, D Flip-Flop3/3, D Flip-Flop1/3, D Flip-Flop7/3
  D Flip-Flop10/2 -> Terminator11/1
  clock/1 -> D Flip-Flop6/2, D Flip-Flop11/2, D Flip-Flop10/2, D Flip-Flop9/2, D Flip-Flop5/2, D Flip-Flop4/2, D Flip-Flop8/2, D Flip-Flop2/2, D Flip-Flop3/2, D Flip-Flop1/2, D Flip-Flop7/2
  alpha/1 -> D Flip-Flop7/1
  Demux/1 -> Switch/1
  Mux/1 -> progressive_mux/1
  Demux/2 -> Switch1/1
  Demux/3 -> Switch2/1
  Demux/4 -> Switch3/1
  Demux/5 -> Switch4/1
  Demux/6 -> Switch5/1
  Demux/7 -> Switch6/1
  Demux/8 -> Switch7/1
  Demux/9 -> Switch8/1
  Demux/10 -> Switch9/1
  Demux/11 -> Switch10/1
  Demux1/1 -> Switch/3
  Demux1/2 -> Switch1/3
  Demux1/3 -> Switch2/3
  Demux1/4 -> Switch3/3
  Demux1/5 -> Switch4/3
  Demux1/6 -> Switch5/3
  Demux1/7 -> Switch6/3
  Demux1/8 -> Switch7/3
  Demux1/9 -> Switch8/3
  Demux1/10 -> Switch9/3
  Demux1/11 -> Switch10/3
  Switch/1 -> Mux/1
  Switch1/1 -> Mux/2
  Switch2/1 -> Mux/3
  Switch3/1 -> Mux/4
  Switch4/1 -> Mux/5
  Switch5/1 -> Mux/6
  Switch6/1 -> Mux/7
  Switch7/1 -> Mux/8
  Switch8/1 -> Mux/9
  Switch9/1 -> Mux/10
  Switch10/1 -> Mux/11

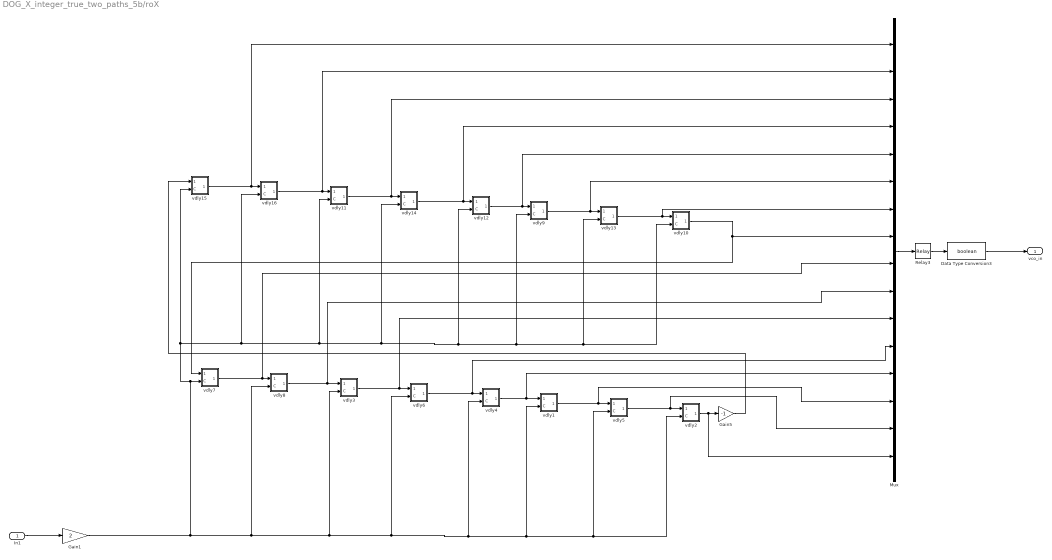
== system DOG_X_integer_true_two_paths_5b/roX ==
  In1 : Inport
  Data Type Conversion3 : DataTypeConversion  OutDataTypeStr=boolean  SaturateOnIntegerOverflow=off  RndMeth=Floor
  Gain1 : Gain  Gain=2
  Gain5 : Gain  Gain=-1
  Mux : Mux  Inputs=16
  Relay3 : Relay
  vdly1 : Subsystem
  vdly10 : Subsystem
  vdly11 : Subsystem
  vdly12 : Subsystem
  vdly13 : Subsystem
  vdly14 : Subsystem
  vdly15 : Subsystem
  vdly16 : Subsystem
  vdly2 : Subsystem
  vdly3 : Subsystem
  vdly4 : Subsystem
  vdly5 : Subsystem
  vdly6 : Subsystem
  vdly7 : Subsystem
  vdly8 : Subsystem
  vdly9 : Subsystem
  vco_in : Outport
  wires:
  vdly2/1(Out) -> Mux/16, Gain5/1
  In1/1 -> Gain1/1
  Gain1/1 -> vdly15/2(C), vdly16/2(C), vdly11/2(C), vdly14/2(C), vdly12/2(C), vdly9/2(C), vdly10/2(C), vdly13/2(C), vdly7/2(C), vdly8/2(C), vdly3/2(C), vdly6/2(C), vdly4/2(C), vdly1/2(C), vdly2/2(C), vdly5/2(C)
  Gain5/1 -> vdly15/1(In)
  Mux/1 -> Relay3/1
  Relay3/1 -> Data Type Conversion3/1
  Data Type Conversion3/1 -> vco_in/1
  vdly5/1(Out) -> Mux/15, vdly2/1(In)
  vdly1/1(Out) -> Mux/14, vdly5/1(In)
  vdly4/1(Out) -> Mux/13, vdly1/1(In)
  vdly6/1(Out) -> Mux/12, vdly4/1(In)
  vdly3/1(Out) -> Mux/11, vdly6/1(In)
  vdly8/1(Out) -> Mux/10, vdly3/1(In)
  vdly7/1(Out) -> vdly8/1(In), Mux/9
  vdly15/1(Out) -> Mux/1, vdly16/1(In)
  vdly16/1(Out) -> Mux/2, vdly11/1(In)
  vdly11/1(Out) -> Mux/3, vdly14/1(In)
  vdly14/1(Out) -> Mux/4, vdly12/1(In)
  vdly12/1(Out) -> Mux/5, vdly9/1(In)
  vdly9/1(Out) -> Mux/6, vdly13/1(In)
  vdly13/1(Out) -> Mux/7, vdly10/1(In)
  vdly10/1(Out) -> vdly7/1(In), Mux/8

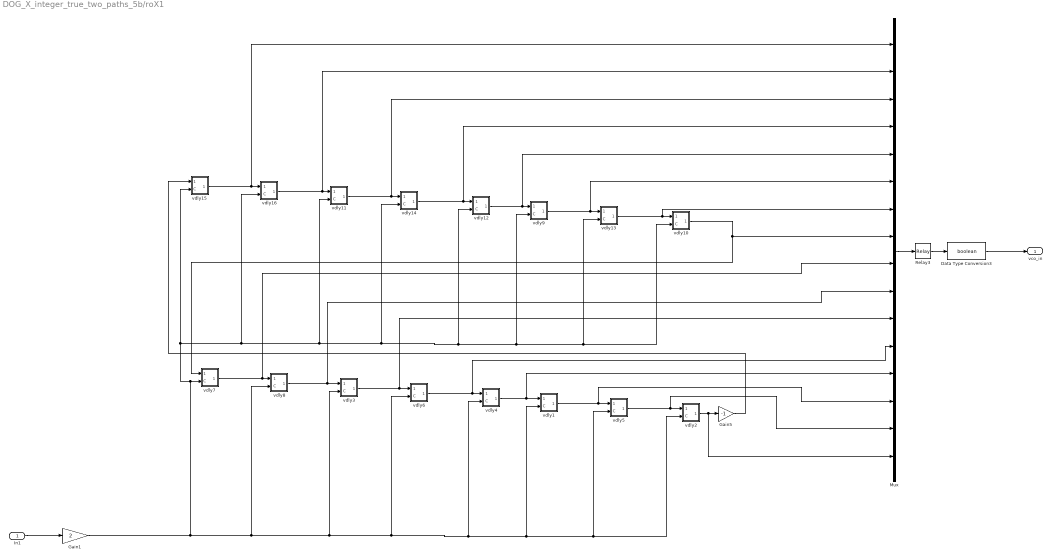
== system DOG_X_integer_true_two_paths_5b/roX1 ==
  In1 : Inport
  Data Type Conversion3 : DataTypeConversion  OutDataTypeStr=boolean  SaturateOnIntegerOverflow=off  RndMeth=Floor
  Gain1 : Gain  Gain=2
  Gain5 : Gain  Gain=-1
  Mux : Mux  Inputs=16
  Relay3 : Relay
  vdly1 : Subsystem
  vdly10 : Subsystem
  vdly11 : Subsystem
  vdly12 : Subsystem
  vdly13 : Subsystem
  vdly14 : Subsystem
  vdly15 : Subsystem
  vdly16 : Subsystem
  vdly2 : Subsystem
  vdly3 : Subsystem
  vdly4 : Subsystem
  vdly5 : Subsystem
  vdly6 : Subsystem
  vdly7 : Subsystem
  vdly8 : Subsystem
  vdly9 : Subsystem
  vco_in : Outport
  wires:
  vdly2/1(Out) -> Mux/16, Gain5/1
  In1/1 -> Gain1/1
  Gain1/1 -> vdly15/2(C), vdly16/2(C), vdly11/2(C), vdly14/2(C), vdly12/2(C), vdly9/2(C), vdly10/2(C), vdly13/2(C), vdly7/2(C), vdly8/2(C), vdly3/2(C), vdly6/2(C), vdly4/2(C), vdly1/2(C), vdly2/2(C), vdly5/2(C)
  Gain5/1 -> vdly15/1(In)
  Mux/1 -> Relay3/1
  Relay3/1 -> Data Type Conversion3/1
  Data Type Conversion3/1 -> vco_in/1
  vdly5/1(Out) -> Mux/15, vdly2/1(In)
  vdly1/1(Out) -> Mux/14, vdly5/1(In)
  vdly4/1(Out) -> Mux/13, vdly1/1(In)
  vdly6/1(Out) -> Mux/12, vdly4/1(In)
  vdly3/1(Out) -> Mux/11, vdly6/1(In)
  vdly8/1(Out) -> Mux/10, vdly3/1(In)
  vdly7/1(Out) -> vdly8/1(In), Mux/9
  vdly15/1(Out) -> Mux/1, vdly16/1(In)
  vdly16/1(Out) -> Mux/2, vdly11/1(In)
  vdly11/1(Out) -> Mux/3, vdly14/1(In)
  vdly14/1(Out) -> Mux/4, vdly12/1(In)
  vdly12/1(Out) -> Mux/5, vdly9/1(In)
  vdly9/1(Out) -> Mux/6, vdly13/1(In)
  vdly13/1(Out) -> Mux/7, vdly10/1(In)
  vdly10/1(Out) -> vdly7/1(In), Mux/8

== system DOG_X_integer_true_two_paths_5b/roX2 ==
  In1 : Inport
  Data Type Conversion3 : DataTypeConversion  OutDataTypeStr=boolean  SaturateOnIntegerOverflow=off  RndMeth=Floor
  Gain1 : Gain  Gain=2
  Gain5 : Gain  Gain=-1
  Mux : Mux  Inputs=16
  Relay3 : Relay
  vdly1 : Subsystem
  vdly10 : Subsystem
  vdly11 : Subsystem
  vdly12 : Subsystem
  vdly13 : Subsystem
  vdly14 : Subsystem
  vdly15 : Subsystem
  vdly16 : Subsystem
  vdly2 : Subsystem
  vdly3 : Subsystem
  vdly4 : Subsystem
  vdly5 : Subsystem
  vdly6 : Subsystem
  vdly7 : Subsystem
  vdly8 : Subsystem
  vdly9 : Subsystem
  vco_in : Outport
  wires:
  vdly2/1(Out) -> Mux/16, Gain5/1
  In1/1 -> Gain1/1
  Gain1/1 -> vdly15/2(C), vdly16/2(C), vdly11/2(C), vdly14/2(C), vdly12/2(C), vdly9/2(C), vdly10/2(C), vdly13/2(C), vdly7/2(C), vdly8/2(C), vdly3/2(C), vdly6/2(C), vdly4/2(C), vdly1/2(C), vdly2/2(C), vdly5/2(C)
  Gain5/1 -> vdly15/1(In)
  Mux/1 -> Relay3/1
  Relay3/1 -> Data Type Conversion3/1
  Data Type Conversion3/1 -> vco_in/1
  vdly5/1(Out) -> Mux/15, vdly2/1(In)
  vdly1/1(Out) -> Mux/14, vdly5/1(In)
  vdly4/1(Out) -> Mux/13, vdly1/1(In)
  vdly6/1(Out) -> Mux/12, vdly4/1(In)
  vdly3/1(Out) -> Mux/11, vdly6/1(In)
  vdly8/1(Out) -> Mux/10, vdly3/1(In)
  vdly7/1(Out) -> vdly8/1(In), Mux/9
  vdly15/1(Out) -> Mux/1, vdly16/1(In)
  vdly16/1(Out) -> Mux/2, vdly11/1(In)
  vdly11/1(Out) -> Mux/3, vdly14/1(In)
  vdly14/1(Out) -> Mux/4, vdly12/1(In)
  vdly12/1(Out) -> Mux/5, vdly9/1(In)
  vdly9/1(Out) -> Mux/6, vdly13/1(In)
  vdly13/1(Out) -> Mux/7, vdly10/1(In)
  vdly10/1(Out) -> vdly7/1(In), Mux/8

== system DOG_X_integer_true_two_paths_5b/roX3 ==
  In1 : Inport
  Data Type Conversion3 : DataTypeConversion  OutDataTypeStr=boolean  SaturateOnIntegerOverflow=off  RndMeth=Floor
  Gain1 : Gain  Gain=2
  Gain5 : Gain  Gain=-1
  Mux : Mux  Inputs=16
  Relay3 : Relay
  vdly1 : Subsystem
  vdly10 : Subsystem
  vdly11 : Subsystem
  vdly12 : Subsystem
  vdly13 : Subsystem
  vdly14 : Subsystem
  vdly15 : Subsystem
  vdly16 : Subsystem
  vdly2 : Subsystem
  vdly3 : Subsystem
  vdly4 : Subsystem
  vdly5 : Subsystem
  vdly6 : Subsystem
  vdly7 : Subsystem
  vdly8 : Subsystem
  vdly9 : Subsystem
  vco_in : Outport
  wires:
  vdly2/1(Out) -> Mux/16, Gain5/1
  In1/1 -> Gain1/1
  Gain1/1 -> vdly15/2(C), vdly16/2(C), vdly11/2(C), vdly14/2(C), vdly12/2(C), vdly9/2(C), vdly10/2(C), vdly13/2(C), vdly7/2(C), vdly8/2(C), vdly3/2(C), vdly6/2(C), vdly4/2(C), vdly1/2(C), vdly2/2(C), vdly5/2(C)
  Gain5/1 -> vdly15/1(In)
  Mux/1 -> Relay3/1
  Relay3/1 -> Data Type Conversion3/1
  Data Type Conversion3/1 -> vco_in/1
  vdly5/1(Out) -> Mux/15, vdly2/1(In)
  vdly1/1(Out) -> Mux/14, vdly5/1(In)
  vdly4/1(Out) -> Mux/13, vdly1/1(In)
  vdly6/1(Out) -> Mux/12, vdly4/1(In)
  vdly3/1(Out) -> Mux/11, vdly6/1(In)
  vdly8/1(Out) -> Mux/10, vdly3/1(In)
  vdly7/1(Out) -> vdly8/1(In), Mux/9
  vdly15/1(Out) -> Mux/1, vdly16/1(In)
  vdly16/1(Out) -> Mux/2, vdly11/1(In)
  vdly11/1(Out) -> Mux/3, vdly14/1(In)
  vdly14/1(Out) -> Mux/4, vdly12/1(In)
  vdly12/1(Out) -> Mux/5, vdly9/1(In)
  vdly9/1(Out) -> Mux/6, vdly13/1(In)
  vdly13/1(Out) -> Mux/7, vdly10/1(In)
  vdly10/1(Out) -> vdly7/1(In), Mux/8

== system DOG_X_integer_true_two_paths_5b/Subsystem/ 2 bit arithmetic left shift ==
  in : Inport
  Constant : Constant  Value=0  OutDataTypeStr=boolean
  Demux1 : Demux  Outputs=9
  Mux : Mux  Inputs=11
  x4 : Outport
  wires:
  Mux/1 -> x4/1
  in/1 -> Demux1/1
  Demux1/1 -> Mux/1
  Demux1/2 -> Mux/2
  Demux1/3 -> Mux/3
  Demux1/4 -> Mux/4
  Demux1/5 -> Mux/5
  Demux1/6 -> Mux/6
  Demux1/7 -> Mux/7
  Demux1/8 -> Mux/8
  Demux1/9 -> Mux/9
  Constant/1 -> Mux/11, Mux/10

== system DOG_X_integer_true_two_paths_5b/Subsystem/ 2 bit extension ==
  in : Inport
  Demux1 : Demux  Outputs=9
  Mux : Mux  Inputs=11
  extended : Outport
  wires:
  Mux/1 -> extended/1
  in/1 -> Demux1/1
  Demux1/1 -> Mux/3, Mux/2, Mux/1
  Demux1/2 -> Mux/4
  Demux1/3 -> Mux/5
  Demux1/4 -> Mux/6
  Demux1/5 -> Mux/7
  Demux1/6 -> Mux/8
  Demux1/7 -> Mux/9
  Demux1/8 -> Mux/10
  Demux1/9 -> Mux/11

== system DOG_X_integer_true_two_paths_5b/Subsystem/2ND_Noise_Shaper_pipelined3 ==
  note: 1 / (2^n_shift)
  Cmux1 : Inport
  Data Type Conversion1 : DataTypeConversion  OutDataTypeStr=fixdt(1,Nbsv2,0)  SaturateOnIntegerOverflow=off  RndMeth=Floor
  Data Type Conversion2 : DataTypeConversion  OutDataTypeStr=fixdt(1,Nbsv2,0)  SaturateOnIntegerOverflow=off  RndMeth=Floor
  Delay4 : Delay  DelayLength=1  SampleTime=Ts
  Gain11 : Gain  Gain=1/2^(Nbsv2-Nbsv1)  OutDataTypeStr=fixdt(1,Nbsv1,0)
  M3 : Delay  DelayLength=1  SampleTime=T2
  M4 : Delay  DelayLength=1  SampleTime=T2
  M5 : ZeroOrderHold  SampleTime=Ts
  Sum20 : Sum  Inputs=|+-  OutDataTypeStr=fixdt(1,Nbsv1,0)
  Sum22 : Sum  Inputs=|+-  OutDataTypeStr=fixdt(1,Nbsv2,0)
  Sum8 : Sum  Inputs=|++  OutDataTypeStr=fixdt(1,Nbsv2,0)
  Y1 : Outport
  Y : Outport  Port=2
  wires:
  M5/1 -> Gain11/1
  Data Type Conversion2/1 -> M3/1
  M3/1 -> Sum8/1
  Sum20/1 -> Data Type Conversion2/1
  Delay4/1 -> Sum22/2
  Sum8/1 -> M4/1
  M4/1 -> Sum8/2, M5/1
  Cmux1/1 -> Sum20/1
  Gain11/1 -> Data Type Conversion1/1
  Sum22/1 -> Y/1
  Data Type Conversion1/1 -> Sum20/2, Y1/1, Sum22/1, Delay4/1

== system DOG_X_integer_true_two_paths_5b/Subsystem/Noise_shaper1 ==
  InP : Inport
  InN : Inport  Port=2
  clock_fast : Inport  Port=3
  clock_slow : Inport  Port=4
  clock_sample : Inport  Port=5
  " 2 bit arithmetic right shift" : Subsystem
  DCO : Subsystem
  differential substraction (9 bit) : Subsystem
  feedback substraction (9 bit) : Subsystem
  first difference substraction (9 bit) : Subsystem
  first difference substraction (9 bit)2 : Subsystem
  register2 : Subsystem
  register3 : Subsystem
  register4 : Subsystem
  register5 : Subsystem
  Y : Outport
  Y1 : Outport  Port=2
  wires:
  " 2 bit arithmetic right shift"/1(9 MSB) -> register4/2(D)
  register4/1(Q) -> first difference substraction (9 bit)/1(plus), feedback substraction (9 bit)/2(minus), register5/2(D)
  feedback substraction (9 bit)/1(subs) -> DCO/2(control)
  DCO/1(output) -> " 2 bit arithmetic right shift"/1(in)
  differential substraction (9 bit)/1(subs) -> register2/2(D), feedback substraction (9 bit)/1(plus)
  clock_fast/1 -> DCO/1(clock)
  clock_slow/1 -> register3/1(CLK), register2/1(CLK)
  register2/1(Q) -> first difference substraction (9 bit)2/1(plus), register3/2(D)
  first difference substraction (9 bit)/1(subs) -> Y/1
  first difference substraction (9 bit)2/1(subs) -> Y1/1
  InP/1 -> differential substraction (9 bit)/1(counter P)
  InN/1 -> differential substraction (9 bit)/2(conter N)
  clock_sample/1 -> register4/1(CLK), register5/1(CLK)
  register3/1(Q) -> first difference substraction (9 bit)2/2(minus)
  register5/1(Q) -> first difference substraction (9 bit)/2(minus)

== system DOG_X_integer_true_two_paths_5b/Subsystem/Noise_shaper2 ==
  InP : Inport
  InN : Inport  Port=2
  clock_fast : Inport  Port=3
  clock_slow : Inport  Port=4
  clock_sample : Inport  Port=5
  " 2 bit arithmetic right shift" : Subsystem
  DCO : Subsystem
  differential substraction (9 bit) : Subsystem
  feedback substraction (9 bit) : Subsystem
  first difference substraction (9 bit) : Subsystem
  first difference substraction (9 bit)2 : Subsystem
  register2 : Subsystem
  register3 : Subsystem
  register4 : Subsystem
  register5 : Subsystem
  Y : Outport
  Y1 : Outport  Port=2
  wires:
  " 2 bit arithmetic right shift"/1(9 MSB) -> register4/2(D)
  register4/1(Q) -> first difference substraction (9 bit)/1(plus), feedback substraction (9 bit)/2(minus), register5/2(D)
  feedback substraction (9 bit)/1(subs) -> DCO/2(control)
  DCO/1(output) -> " 2 bit arithmetic right shift"/1(in)
  differential substraction (9 bit)/1(subs) -> register2/2(D), feedback substraction (9 bit)/1(plus)
  clock_fast/1 -> DCO/1(clock)
  clock_slow/1 -> register3/1(CLK), register2/1(CLK)
  register2/1(Q) -> first difference substraction (9 bit)2/1(plus), register3/2(D)
  first difference substraction (9 bit)/1(subs) -> Y/1
  first difference substraction (9 bit)2/1(subs) -> Y1/1
  InP/1 -> differential substraction (9 bit)/1(counter P)
  InN/1 -> differential substraction (9 bit)/2(conter N)
  clock_sample/1 -> register4/1(CLK), register5/1(CLK)
  register3/1(Q) -> first difference substraction (9 bit)2/2(minus)
  register5/1(Q) -> first difference substraction (9 bit)/2(minus)

== system DOG_X_integer_true_two_paths_5b/Subsystem/mux ==
  data_HDR : Inport
  data_HSNR : Inport  Port=2
  alpha : Inport  Port=3
  Demux : Demux  Outputs=11
  Demux1 : Demux  Outputs=11
  Mux : Mux  Inputs=11
  Switch{,1..10} (11 alike) : Switch  Criteria=u2 > Threshold  SaturateOnIntegerOverflow=off  InputSameDT=off
  out : Outport
  wires:
  alpha/1 -> Switch1/2, Switch2/2, Switch3/2, Switch4/2, Switch6/2, Switch7/2, Switch8/2, Switch9/2, Switch10/2, Switch5/2, Switch/2
  data_HDR/1 -> Demux/1
  data_HSNR/1 -> Demux1/1
  Demux/1 -> Switch/1
  Mux/1 -> out/1
  Demux/2 -> Switch1/1
  Demux/3 -> Switch2/1
  Demux/4 -> Switch3/1
  Demux/5 -> Switch4/1
  Demux/6 -> Switch5/1
  Demux/7 -> Switch6/1
  Demux/8 -> Switch7/1
  Demux/9 -> Switch8/1
  Demux/10 -> Switch9/1
  Demux/11 -> Switch10/1
  Demux1/1 -> Switch/3
  Demux1/2 -> Switch1/3
  Demux1/3 -> Switch2/3
  Demux1/4 -> Switch3/3
  Demux1/5 -> Switch4/3
  Demux1/6 -> Switch5/3
  Demux1/7 -> Switch6/3
  Demux1/8 -> Switch7/3
  Demux1/9 -> Switch8/3
  Demux1/10 -> Switch9/3
  Demux1/11 -> Switch10/3
  Switch/1 -> Mux/1
  Switch1/1 -> Mux/2
  Switch2/1 -> Mux/3
  Switch3/1 -> Mux/4
  Switch4/1 -> Mux/5
  Switch5/1 -> Mux/6
  Switch6/1 -> Mux/7
  Switch7/1 -> Mux/8
  Switch8/1 -> Mux/9
  Switch9/1 -> Mux/10
  Switch10/1 -> Mux/11

== system DOG_X_integer_true_two_paths_5b/Subsystem/mux1 ==
  progressive : Inport
  non_progressive : Inport  Port=2
  select : Inport  Port=3
  Demux : Demux  Outputs=11
  Demux1 : Demux  Outputs=11
  Mux : Mux  Inputs=11
  Switch{,1..10} (11 alike) : Switch  Criteria=u2 > Threshold  SaturateOnIntegerOverflow=off  InputSameDT=off
  out : Outport
  wires:
  select/1 -> Switch1/2, Switch2/2, Switch3/2, Switch4/2, Switch6/2, Switch7/2, Switch8/2, Switch9/2, Switch10/2, Switch5/2, Switch/2
  progressive/1 -> Demux/1
  non_progressive/1 -> Demux1/1
  Demux/1 -> Switch/1
  Mux/1 -> out/1
  Demux/2 -> Switch1/1
  Demux/3 -> Switch2/1
  Demux/4 -> Switch3/1
  Demux/5 -> Switch4/1
  Demux/6 -> Switch5/1
  Demux/7 -> Switch6/1
  Demux/8 -> Switch7/1
  Demux/9 -> Switch8/1
  Demux/10 -> Switch9/1
  Demux/11 -> Switch10/1
  Demux1/1 -> Switch/3
  Demux1/2 -> Switch1/3
  Demux1/3 -> Switch2/3
  Demux1/4 -> Switch3/3
  Demux1/5 -> Switch4/3
  Demux1/6 -> Switch5/3
  Demux1/7 -> Switch6/3
  Demux1/8 -> Switch7/3
  Demux1/9 -> Switch8/3
  Demux1/10 -> Switch9/3
  Demux1/11 -> Switch10/3
  Switch/1 -> Mux/1
  Switch1/1 -> Mux/2
  Switch2/1 -> Mux/3
  Switch3/1 -> Mux/4
  Switch4/1 -> Mux/5
  Switch5/1 -> Mux/6
  Switch6/1 -> Mux/7
  Switch7/1 -> Mux/8
  Switch8/1 -> Mux/9
  Switch9/1 -> Mux/10
  Switch10/1 -> Mux/11

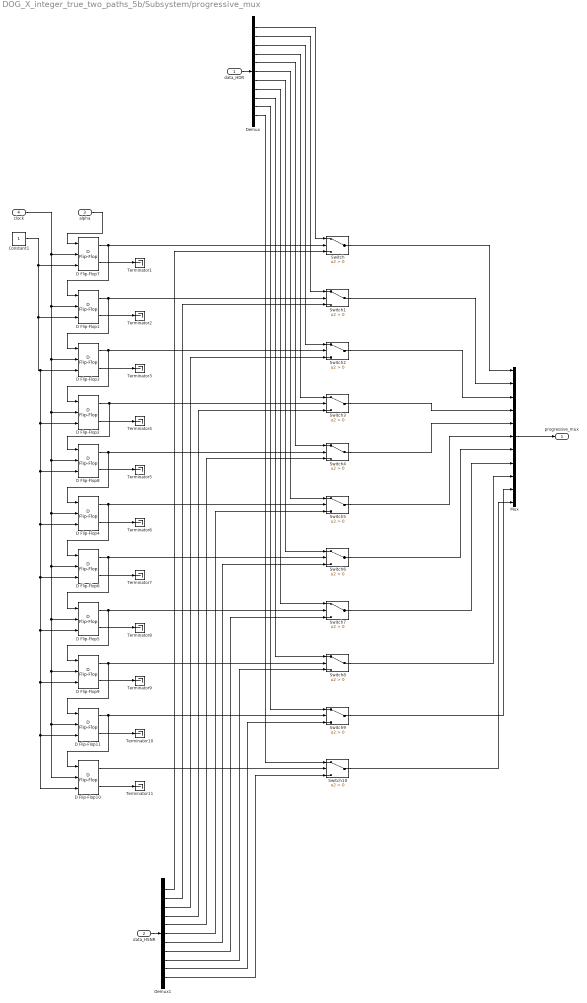
== system DOG_X_integer_true_two_paths_5b/Subsystem/progressive_mux ==
  data_HDR : Inport
  data_HSNR : Inport  Port=2
  alpha : Inport  Port=3
  clock : Inport  Port=4
  Constant1 : Constant  OutDataTypeStr=boolean
  D Flip-Flop{1..11} (11 alike) : simulink_extras/Flip Flops/D Flip-Flop
  Demux : Demux  Outputs=11
  Demux1 : Demux  Outputs=11
  Mux : Mux  Inputs=11
  Switch{,1..10} (11 alike) : Switch  Criteria=u2 > Threshold  SaturateOnIntegerOverflow=off  InputSameDT=off
  Terminator{1..11} (11 alike) : Terminator
  progressive_mux : Outport
  wires:
  D Flip-Flop7/1 -> Switch/2, D Flip-Flop1/1
  data_HDR/1 -> Demux/1
  data_HSNR/1 -> Demux1/1
  D Flip-Flop7/2 -> Terminator1/1
  D Flip-Flop1/2 -> Terminator2/1
  D Flip-Flop1/1 -> D Flip-Flop3/1, Switch1/2
  D Flip-Flop3/1 -> Switch2/2, D Flip-Flop2/1
  D Flip-Flop2/2 -> Terminator4/1
  D Flip-Flop3/2 -> Terminator3/1
  D Flip-Flop2/1 -> Switch3/2, D Flip-Flop8/1
  D Flip-Flop4/2 -> Terminator6/1
  D Flip-Flop8/1 -> Switch4/2, D Flip-Flop4/1
  D Flip-Flop6/2 -> Terminator7/1
  D Flip-Flop5/2 -> Terminator8/1
  D Flip-Flop6/1 -> Switch6/2, D Flip-Flop5/1
  D Flip-Flop8/2 -> Terminator5/1
  D Flip-Flop4/1 -> D Flip-Flop6/1, Switch5/2
  D Flip-Flop11/1 -> Switch9/2, D Flip-Flop10/1
  D Flip-Flop9/1 -> D Flip-Flop11/1, Switch8/2
  D Flip-Flop5/1 -> D Flip-Flop9/1, Switch7/2
  D Flip-Flop9/2 -> Terminator9/1
  D Flip-Flop11/2 -> Terminator10/1
  D Flip-Flop10/1 -> Switch10/2
  Constant1/1 -> D Flip-Flop8/3, D Flip-Flop10/3, D Flip-Flop11/3, D Flip-Flop9/3, D Flip-Flop5/3, D Flip-Flop6/3, D Flip-Flop4/3, D Flip-Flop2/3, D Flip-Flop3/3, D Flip-Flop1/3, D Flip-Flop7/3
  D Flip-Flop10/2 -> Terminator11/1
  clock/1 -> D Flip-Flop6/2, D Flip-Flop11/2, D Flip-Flop10/2, D Flip-Flop9/2, D Flip-Flop5/2, D Flip-Flop4/2, D Flip-Flop8/2, D Flip-Flop2/2, D Flip-Flop3/2, D Flip-Flop1/2, D Flip-Flop7/2
  alpha/1 -> D Flip-Flop7/1
  Demux/1 -> Switch/1
  Mux/1 -> progressive_mux/1
  Demux/2 -> Switch1/1
  Demux/3 -> Switch2/1
  Demux/4 -> Switch3/1
  Demux/5 -> Switch4/1
  Demux/6 -> Switch5/1
  Demux/7 -> Switch6/1
  Demux/8 -> Switch7/1
  Demux/9 -> Switch8/1
  Demux/10 -> Switch9/1
  Demux/11 -> Switch10/1
  Demux1/1 -> Switch/3
  Demux1/2 -> Switch1/3
  Demux1/3 -> Switch2/3
  Demux1/4 -> Switch3/3
  Demux1/5 -> Switch4/3
  Demux1/6 -> Switch5/3
  Demux1/7 -> Switch6/3
  Demux1/8 -> Switch7/3
  Demux1/9 -> Switch8/3
  Demux1/10 -> Switch9/3
  Demux1/11 -> Switch10/3
  Switch/1 -> Mux/1
  Switch1/1 -> Mux/2
  Switch2/1 -> Mux/3
  Switch3/1 -> Mux/4
  Switch4/1 -> Mux/5
  Switch5/1 -> Mux/6
  Switch6/1 -> Mux/7
  Switch7/1 -> Mux/8
  Switch8/1 -> Mux/9
  Switch9/1 -> Mux/10
  Switch10/1 -> Mux/11

== system DOG_X_integer_true_two_paths_5b/Subsystem/substractor2 ==
  note: to 2's comp (NbC1 bits)
  C2p : Inport
  C2n : Inport  Port=2
  Add1 : Sum
  Add2 : Sum
  Constant13 : Constant  Value=-(2^(Nbsv1-1))
  Data Type Conversion : DataTypeConversion  OutDataTypeStr=fixdt(1,Nbsv1,0)  SaturateOnIntegerOverflow=off  RndMeth=Floor
  Data Type Conversion1 : DataTypeConversion  OutDataTypeStr=fixdt(1,Nbsv1,0)  SaturateOnIntegerOverflow=off  RndMeth=Floor
  M2 : Delay  DelayLength=1  SampleTime=T2
  Sum19 : Sum  Inputs=+-  OutDataTypeStr=fixdt(1,Nbsv1,0)
  Cmux1 : Outport
  wires:
  Data Type Conversion1/1 -> Sum19/2
  Add1/1 -> Data Type Conversion/1
  Constant13/1 -> Add2/1, Add1/1
  Data Type Conversion/1 -> Sum19/1
  Sum19/1 -> M2/1
  Add2/1 -> Data Type Conversion1/1
  C2p/1 -> Add1/2
  M2/1 -> Cmux1/1
  C2n/1 -> Add2/2

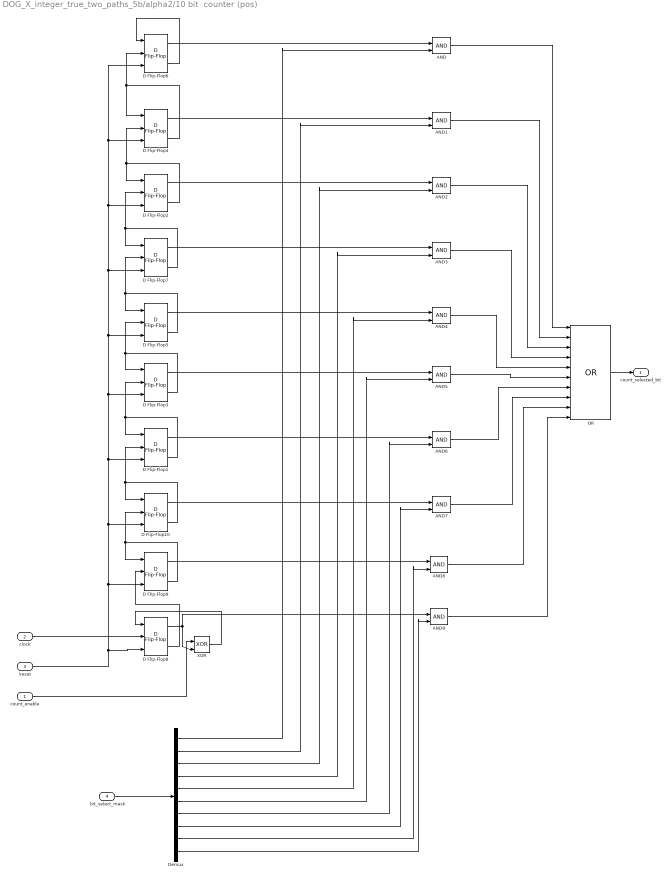
== system DOG_X_integer_true_two_paths_5b/alpha2/10 bit  counter (pos) ==
  count_enable : Inport
  clock : Inport  Port=2
  !reset : Inport  Port=3
  bit_select_mask : Inport  Port=4
  AND{,1..9} (10 alike) : Logic  IconShape=distinctive  AllPortsSameDT=off  OutDataTypeStr=boolean
  D Flip-Flop{1..10} (10 alike) : simulink_extras/Flip Flops/D Flip-Flop
  Demux : Demux  Outputs=10
  OR : Logic  Operator=OR  Inputs=10  IconShape=distinctive  AllPortsSameDT=off  OutDataTypeStr=boolean
  XOR : Logic  Operator=XOR  IconShape=distinctive  AllPortsSameDT=off  OutDataTypeStr=boolean
  count_selected_bit : Outport
  wires:
  D Flip-Flop1/2 -> D Flip-Flop3/2, D Flip-Flop1/1
  D Flip-Flop3/2 -> D Flip-Flop3/1, D Flip-Flop5/2
  D Flip-Flop5/2 -> D Flip-Flop7/2, D Flip-Flop5/1
  D Flip-Flop7/2 -> D Flip-Flop2/2, D Flip-Flop7/1
  D Flip-Flop2/2 -> D Flip-Flop4/2, D Flip-Flop2/1
  D Flip-Flop4/2 -> D Flip-Flop6/2, D Flip-Flop4/1
  D Flip-Flop6/2 -> D Flip-Flop6/1
  D Flip-Flop9/2 -> D Flip-Flop9/1, D Flip-Flop10/2
  D Flip-Flop10/2 -> D Flip-Flop1/2, D Flip-Flop10/1
  !reset/1 -> D Flip-Flop8/3, D Flip-Flop9/3, D Flip-Flop10/3, D Flip-Flop3/3, D Flip-Flop5/3, D Flip-Flop6/3, D Flip-Flop4/3, D Flip-Flop2/3, D Flip-Flop7/3, D Flip-Flop1/3
  clock/1 -> D Flip-Flop8/2
  D Flip-Flop8/2 -> D Flip-Flop9/2
  count_enable/1 -> XOR/1
  XOR/1 -> D Flip-Flop8/1
  D Flip-Flop4/1 -> AND1/1
  D Flip-Flop2/1 -> AND2/1
  D Flip-Flop7/1 -> AND3/1
  D Flip-Flop5/1 -> AND4/1
  D Flip-Flop1/1 -> AND6/1
  D Flip-Flop10/1 -> AND7/1
  D Flip-Flop9/1 -> AND8/1
  D Flip-Flop8/1 -> AND9/1, XOR/2
  D Flip-Flop6/1 -> AND/1
  OR/1 -> count_selected_bit/1
  bit_select_mask/1 -> Demux/1
  D Flip-Flop3/1 -> AND5/1
  AND/1 -> OR/1
  AND1/1 -> OR/2
  AND2/1 -> OR/3
  AND3/1 -> OR/4
  AND4/1 -> OR/5
  AND5/1 -> OR/6
  AND6/1 -> OR/7
  AND7/1 -> OR/8
  AND8/1 -> OR/9
  AND9/1 -> OR/10
  Demux/10 -> AND9/2
  Demux/9 -> AND8/2
  Demux/8 -> AND7/2
  Demux/7 -> AND6/2
  Demux/6 -> AND5/2
  Demux/5 -> AND4/2
  Demux/4 -> AND3/2
  Demux/3 -> AND2/2
  Demux/2 -> AND1/2
  Demux/1 -> AND/2

== system DOG_X_integer_true_two_paths_5b/alpha2/abs ==
  input : Inport
  Constant : Constant  OutDataTypeStr=boolean
  Constant2 : Constant  Value=0  OutDataTypeStr=boolean
  Demux1 : Demux  Outputs=9
  FA10 : Subsystem
  FA2 : Subsystem
  FA3 : Subsystem
  FA4 : Subsystem
  FA5 : Subsystem
  FA6 : Subsystem
  FA7 : Subsystem
  FA9 : Subsystem
  Mux : Mux  Inputs=9
  XOR{,1..7} (8 alike) : Logic  Operator=XOR  IconShape=distinctive  AllPortsSameDT=off  OutDataTypeStr=boolean
  abs(input) : Outport
  wires:
  Mux/1 -> abs(input)/1
  input/1 -> Demux1/1
  FA7/2(Co) -> FA6/3(Cin)
  FA6/2(Co) -> FA5/3(Cin)
  FA5/2(Co) -> FA4/3(Cin)
  FA4/2(Co) -> FA3/3(Cin)
  FA3/2(Co) -> FA2/3(Cin)
  FA9/2(Co) -> FA7/3(Cin)
  FA10/2(Co) -> FA9/2(Cin)
  Constant/1 -> FA10/3(Cin)
  FA2/1(S) -> Mux/2
  FA2/2(Co) -> Mux/1
  FA3/1(S) -> Mux/3
  FA4/1(S) -> Mux/4
  FA5/1(S) -> Mux/5
  FA6/1(S) -> Mux/6
  FA7/1(S) -> Mux/7
  FA9/1(S) -> Mux/8
  FA10/1(S) -> Mux/9
  XOR/1 -> FA2/1(B0)
  Constant2/1 -> FA5/2(B1), FA6/2(B1), FA9/3(B1), FA10/2(B1), FA7/2(B1), FA4/2(B1), FA3/2(B1), FA2/2(B1)
  XOR1/1 -> FA3/1(B0)
  XOR2/1 -> FA4/1(B0)
  XOR3/1 -> FA5/1(B0)
  XOR4/1 -> FA6/1(B0)
  XOR5/1 -> FA7/1(B0)
  XOR6/1 -> FA9/1(B0)
  XOR7/1 -> FA10/1(B0)
  Demux1/1 -> XOR1/1, XOR3/1, XOR4/1, XOR5/1, XOR6/1, XOR7/1, XOR2/1, XOR/1
  Demux1/2 -> XOR/2
  Demux1/3 -> XOR1/2
  Demux1/4 -> XOR2/2
  Demux1/5 -> XOR3/2
  Demux1/6 -> XOR4/2
  Demux1/7 -> XOR5/2
  Demux1/8 -> XOR6/2
  Demux1/9 -> XOR7/2

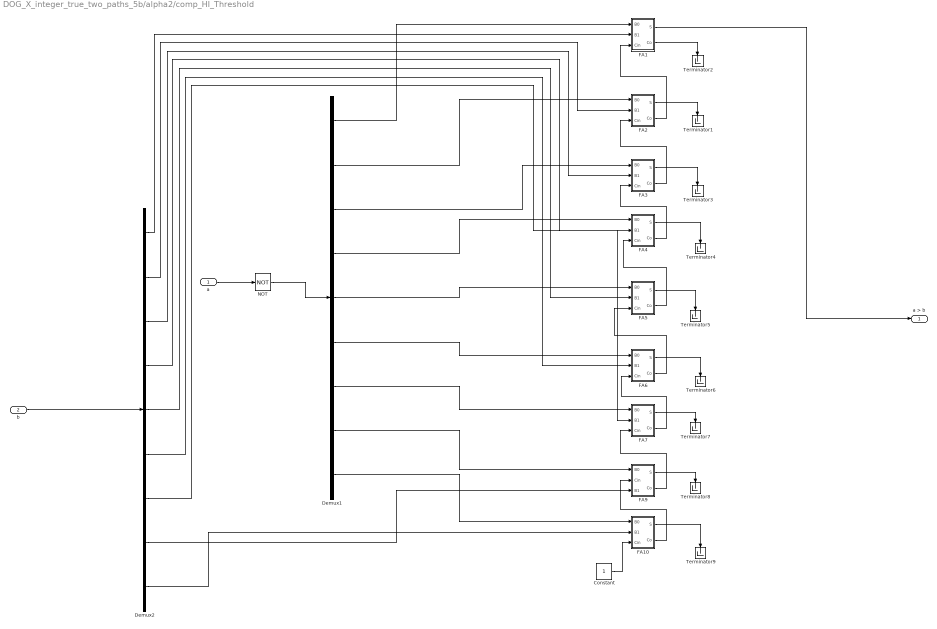
== system DOG_X_integer_true_two_paths_5b/alpha2/comp_HI_Threshold ==
  a : Inport
  b : Inport  Port=2
  Constant : Constant  OutDataTypeStr=boolean
  Demux1 : Demux  Outputs=9
  Demux2 : Demux  Outputs=9
  FA1 : Subsystem
  FA10 : Subsystem
  FA2 : Subsystem
  FA3 : Subsystem
  FA4 : Subsystem
  FA5 : Subsystem
  FA6 : Subsystem
  FA7 : Subsystem
  FA9 : Subsystem
  NOT : Logic  Operator=NOT  IconShape=distinctive  AllPortsSameDT=off  OutDataTypeStr=boolean
  Terminator{1..9} (9 alike) : Terminator
  a > b : Outport
  wires:
  a/1 -> NOT/1
  FA7/2(Co) -> FA6/3(Cin)
  FA6/2(Co) -> FA5/3(Cin)
  FA5/2(Co) -> FA4/3(Cin)
  FA4/2(Co) -> FA3/3(Cin)
  FA3/2(Co) -> FA2/3(Cin)
  FA2/2(Co) -> FA1/3(Cin)
  FA9/2(Co) -> FA7/3(Cin)
  FA10/2(Co) -> FA9/2(Cin)
  Constant/1 -> FA10/3(Cin)
  FA1/2(Co) -> Terminator2/1
  Demux1/9 -> FA10/1(B0)
  Demux1/8 -> FA9/1(B0)
  Demux1/7 -> FA7/1(B0)
  Demux1/6 -> FA6/1(B0)
  Demux1/5 -> FA5/1(B0)
  Demux1/4 -> FA4/1(B0)
  Demux1/2 -> FA2/1(B0)
  Demux1/3 -> FA3/1(B0)
  Demux1/1 -> FA1/1(B0)
  FA1/1(S) -> a > b/1
  Demux2/5 -> FA5/2(B1)
  Demux2/6 -> FA6/2(B1)
  Demux2/1 -> FA1/2(B1)
  Demux2/3 -> FA3/2(B1)
  Demux2/4 -> FA4/2(B1)
  Demux2/2 -> FA2/2(B1)
  Demux2/7 -> FA7/2(B1)
  Demux2/9 -> FA10/2(B1)
  Demux2/8 -> FA9/3(B1)
  FA2/1(S) -> Terminator1/1
  FA3/1(S) -> Terminator3/1
  FA4/1(S) -> Terminator4/1
  FA5/1(S) -> Terminator5/1
  FA6/1(S) -> Terminator6/1
  FA7/1(S) -> Terminator7/1
  FA9/1(S) -> Terminator8/1
  FA10/1(S) -> Terminator9/1
  b/1 -> Demux2/1
  NOT/1 -> Demux1/1
